simulink model "overlab_add"  (R2016a)
settings: Solver=VariableStepAuto  StartTime=0.0  StopTime=1  RelTol=1e-3
undefined symbols (not defined in the file): h1
libraries: dspxfrm3 x3, dspsigops x3, dspmtrx3 x2, dspbuff3 x1
settings Model: Creator=moham  LastModifiedBy=moham

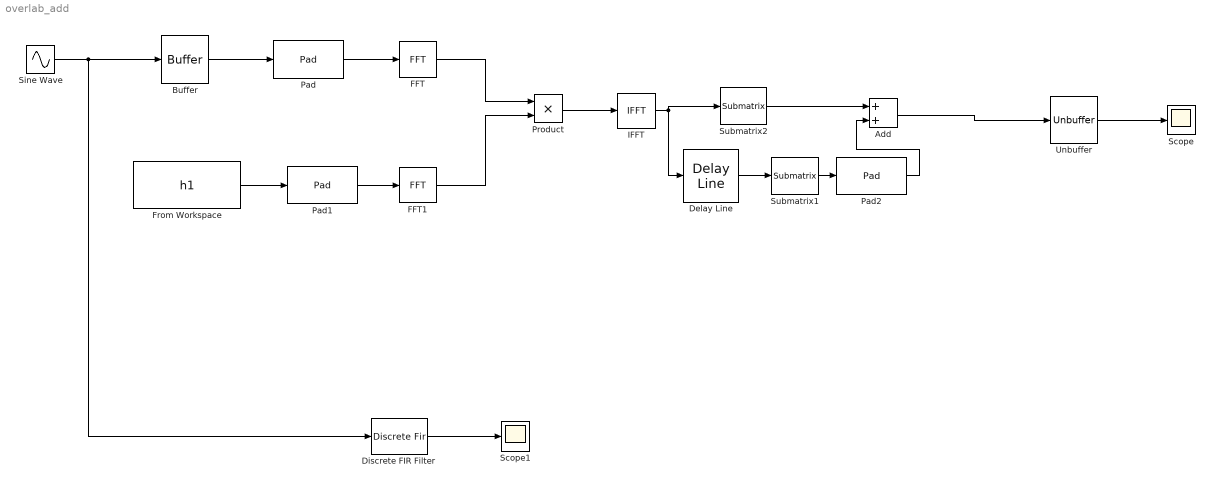
== system overlab_add ==
  Add : Sum
  Buffer : Buffer  N=1548  TreatMby1Signals=One channel  OutputFrames=off
  Delay Line : dspbuff3/Delay Line  siz=2048  ic=0  directfeed=off  enable_output=off  hold_output=off  TreatMby1Signals=One channel  OutputFrames=off
  Discrete FIR Filter : DiscreteFir  Coefficients=h1
  FFT : dspxfrm3/FFT  FFTImplementation=Auto  CompMethod=Table lookup  TableOpt=NEW  TableOptActive=Speed  BitRevOrder=off  Normalize=off  InheritFFTLength=on  FFTLength=64  WrapInput=on  roundingMode=Floor  overflowMode=off  firstCoeffDataTypeStr=Inherit: Same word length as input  firstCoeffLastDataTypeStr=Inherit: Same word length as input  outputMin=[]  outputMax=[]
  FFT1 : dspxfrm3/FFT  FFTImplementation=Auto  CompMethod=Table lookup  TableOpt=NEW  TableOptActive=Speed  BitRevOrder=off  Normalize=off  InheritFFTLength=on  FFTLength=64  WrapInput=on  roundingMode=Floor  overflowMode=off  firstCoeffDataTypeStr=Inherit: Same word length as input  firstCoeffLastDataTypeStr=Inherit: Same word length as input  outputMin=[]  outputMax=[]
  From Workspace : FromWorkspace  VariableName=h1  SampleTime=1548/8000
  IFFT : dspxfrm3/IFFT  FFTImplementation=Auto  CompMethod=Table lookup  TableOpt=NEW  TableOptActive=Speed  BitRevOrder=off  cs_in=off  Normalize=on  InheritFFTLength=on  FFTLength=64  WrapInput=on  mode=Complex  outSamplingMode=Sample based  roundingMode=Floor  overflowMode=off  firstCoeffDataTypeStr=Inherit: Same word length as input  firstCoeffLastDataTypeStr=Inherit: Same word length as input  outputMin=[]  outputMax=[]
  Pad : dspsigops/Pad  padAlong=Columns  dimsToPad=1  valSrc=Specify via dialog  padVal=0  spec=Output size  padNumOutRowsSpecMethod=User-specified  numOutRows=2048  padNumOutColsSpecMethod=User-specified  numOutCols=1  isVarDimsMode=off  padBeginning=0  padEnd=0  outSizeMode=User-specified  outSize=1  padSigAt=End  trunc_flag=None  roundingMode=Floor  overflowMode=off  truncOrWrapMode=Truncate  wrap_flag=None
  Pad1 : dspsigops/Pad  padAlong=Columns  dimsToPad=1  valSrc=Specify via dialog  padVal=0  spec=Output size  padNumOutRowsSpecMethod=User-specified  numOutRows=2048  padNumOutColsSpecMethod=User-specified  numOutCols=1  isVarDimsMode=off  padBeginning=0  padEnd=0  outSizeMode=User-specified  outSize=1  padSigAt=End  trunc_flag=None  roundingMode=Floor  overflowMode=off  truncOrWrapMode=Truncate  wrap_flag=None
  Pad2 : dspsigops/Pad  padAlong=Columns  dimsToPad=1  valSrc=Specify via dialog  padVal=0  spec=Output size  padNumOutRowsSpecMethod=User-specified  numOutRows=1548  padNumOutColsSpecMethod=User-specified  numOutCols=1  isVarDimsMode=off  padBeginning=0  padEnd=0  outSizeMode=User-specified  outSize=1  padSigAt=End  trunc_flag=None  roundingMode=Floor  overflowMode=off  truncOrWrapMode=Truncate  wrap_flag=None
  Product : Product
  Scope : Scope
  Scope1 : Scope
  Sine Wave : Sin  Frequency=200*pi  SampleTime=1/8000
  Submatrix1 : dspmtrx3/Submatrix  RowSpan=Range of rows  RowStartMode=Index  RowStartIndex=1549  RowEndMode=Last  RowEndIndex=1  ColSpan=All columns  ColStartMode=First  ColStartIndex=1  ColEndMode=Last  ColEndIndex=1
  Submatrix2 : dspmtrx3/Submatrix  RowSpan=Range of rows  RowStartMode=First  RowStartIndex=1549  RowEndMode=Index  RowEndIndex=1548  ColSpan=All columns  ColStartMode=First  ColStartIndex=1  ColEndMode=Last  ColEndIndex=1
  Unbuffer : Unbuffer  SampleBasedProcessing=Same as frame based
  wires:
  Sine Wave/1 -> Discrete FIR Filter/1, Buffer/1
  Buffer/1 -> Pad/1
  From Workspace/1 -> Pad1/1
  Pad/1 -> FFT/1
  Pad1/1 -> FFT1/1
  FFT/1 -> Product/1
  FFT1/1 -> Product/2
  Product/1 -> IFFT/1
  IFFT/1 -> Delay Line/1, Submatrix2/1
  Delay Line/1 -> Submatrix1/1
  Unbuffer/1 -> Scope/1
  Submatrix1/1 -> Pad2/1
  Pad2/1 -> Add/2
  Add/1 -> Unbuffer/1
  Submatrix2/1 -> Add/1
  Discrete FIR Filter/1 -> Scope1/1
